simulink model "UAV_sync_unknown_sim"  (R2018b)
settings: Solver=ode23tb  StartTime=0.0  StopTime=35  RelTol=1e-3
values from neighbouring files (symbols this model uses):
  Bm = [zeros(6,6); eye(6)]    [UAV_sync_unknown.m]    (also in UAV_sync_unknown_gap.m)
  C_rho = 1.225    [SC42120_UAV_Preconditions.m]
  D0 = [M0 0 0 0 0 0 ... (first row only)    [SC42120_UAV_Preconditions.m]
  Derivative_gain_phi = 50    [SC42120_UAV_Preconditions.m]
  Derivative_gain_psi = 50    [SC42120_UAV_Preconditions.m]
  Derivative_gain_theta = 50    [SC42120_UAV_Preconditions.m]
  Derivative_gain_x = 50    [SC42120_UAV_Preconditions.m]
  Derivative_gain_y = 50    [SC42120_UAV_Preconditions.m]
  Derivative_gain_z = 50    [SC42120_UAV_Preconditions.m]
  G = 9.80665    [SC42120_UAV_Preconditions.m]
  g0 = [0;0;-M0*G;0;0;0]    [SC42120_UAV_Preconditions.m]
  I0 = [0.02 0 -0.01 ... (first row only)    [SC42120_UAV_Preconditions.m]
  InitWind = [0;0;0]    [SC42120_UAV_Preconditions.m]
  Kp = diag(P)    [SC42120_UAV_Preconditions.m]
  Kv = diag(V)    [SC42120_UAV_Preconditions.m]
  M0 = 10    [SC42120_UAV_Preconditions.m]
  M1 = 20    [UAV_sync_known.m]    (also in UAV_sync_unknown.m; UAV_sync_unknown_gap.m)
  M2 = 30    [UAV_sync_known.m]    (also in UAV_sync_unknown.m; UAV_sync_unknown_gap.m)
  M3 = 40    [UAV_sync_known.m]    (also in UAV_sync_unknown.m; UAV_sync_unknown_gap.m)
  M4 = 50    [UAV_sync_known.m]    (also in UAV_sync_unknown.m; UAV_sync_unknown_gap.m)
  P = [Proportional_x Proportional_y Proportional_z Proportional_phi Proportional_theta Proportional_psi]    [SC42120_UAV_Preconditions.m]    (also in UAV_sync_unknown.m = lyap(Am',Q); UAV_sync_unknown_gap.m = lyap(Am',Q); drawDATCOMaircraft.m = temparray)
  Proportional_phi = 50    [SC42120_UAV_Preconditions.m]
  Proportional_psi = 50    [SC42120_UAV_Preconditions.m]
  Proportional_theta = 50    [SC42120_UAV_Preconditions.m]
  Proportional_x = 50    [SC42120_UAV_Preconditions.m]
  Proportional_y = 50    [SC42120_UAV_Preconditions.m]
  Proportional_z = 50    [SC42120_UAV_Preconditions.m]
undefined symbols (not defined in the file or in its folder): Aero, APlane, Bxl, C, Ctr, deg, DiscIntNeverNeededParam, F, Guid, Init, Light, MIL, Path, rad, s, Trim, Utility
libraries: aerolibconvert2 x37, sharedutil x18, simulink x15, dspsigops x7, shared6dof x6, aerolibasang x4, simulink_extras x3, aerolibadyn x1, aerolibtransform2 x1, aerolibwind2 x1
(part 3 of 7)

== system UAV_sync_unknown_sim/Node 0/VF Approach/AUTOPILOT/Navigation Controller ==
  note: Activate bias only if you have troubles with undesired settling orbits.
  ReferenceCourse : Inport  Unit=deg
  DerCond : Inport  Port=2
  Angle Conversion : aerolibconvert2/Angle Conversion  IU=rad  OU=deg
  Bias : Bias  Bias=360
  Bus Selector : BusSelector  OutputSignals=Course
  Constant : Constant  Value=45
  Discrete PID Controller : simulink/Continuous/PID Controller  Controller=PD  Form=Parallel  TimeDomain=Discrete-time  SampleTime=Ctr.TS  IntegratorMethod=Forward Euler  FilterMethod=Forward Euler  ControllerParametersSource=internal  P=Ctr.Hdg2Roll.NAV_ROLL_P  I=0.01  D=Ctr.Hdg2Roll.NAV_ROLL_D  UseFilter=on  N=2*pi*20  TunerSelectOption=Transfer Function Based (PID Tuner App)  InitialConditionSource=internal  InitialConditionForIntegrator=0  InitialConditionForFilter=0  DifferentiatorICPrevScaledInput=0  ExternalReset=none  TrackingMode=off  Kt=1  LimitOutput=on  UpperSaturationLimit=45  LowerSaturationLimit=-45  LinearizeAsGain=off  AntiWindupMode=clamping  Kb=1  POutMin=[]  POutMax=[]  IOutMin=[]  IOutMax=[]  DOutMin=[]  DOutMax=[]  NOutMin=[]  NOutMax=[]  SumOutMin=[]  SumOutMax=[]  SaturationOutMin=[]  SaturationOutMax=[]  PParamMin=[]  PParamMax=[]  IParamMin=[]  IParamMax=[]  DParamMin=[]  DParamMax=[]  NParamMin=[]  NParamMax=[]  KbParamMin=[]  KbParamMax=[]  KtParamMin=[]  KtParamMax=[]  KbOutMin=[]  KbOutMax=[]  KtOutMin=[]  KtOutMax=[]  IntegratorOutMin=[]  IntegratorOutMax=[]  FilterOutMin=[]  FilterOutMax=[]  SumI1OutMin=[]  SumI1OutMax=[]  SumI2OutMin=[]  SumI2OutMax=[]  SumI3OutMin=[]  SumI3OutMax=[]  SumI4OutMin=[]  SumI4OutMax=[]  SumDOutMin=[]  SumDOutMax=[]  DifferentiatorOutMin=[]  DifferentiatorOutMax=[]  FilterDiffOutCoefMin=[]  FilterDiffOutCoefMax=[]  ReciprocalOutMin=[]  ReciprocalOutMax=[]  SumDenOutMin=[]  SumDenOutMax=[]  SumNumOutMin=[]  SumNumOutMax=[]  DivideOutMin=[]  DivideOutMax=[]  IntegratorContinuousStateAttributes=''  IntegratorStateMustResolveToSignalObject=off  IntegratorRTWStateStorageClass=Auto  FilterContinuousStateAttributes=''  FilterStateMustResolveToSignalObject=off  FilterRTWStateStorageClass=Auto  ParallelPVariant=InternalParameters  IdealPVariant=Disabled  IVariant=Disabled  DVariant=InternalParameters  IntegratorVariant=Disabled  SatVariant=Enabled  AWVariant=Disabled  PCopyVariant=Disabled  TRVariant=Disabled  FdbkBlocksVariant=Forward  IdealPFdbkVariant=Disabled  SatFdbkVariant=Disabled  DerivativeFilterVariant=ForwardEulerFilter  NVariant=InternalParameters  NCopyVariant=Disabled  FilterICVariant=InternalICsFilter  IntegratorICVariant=Disabled  ExternalResetVariant=Disabled  TRSumVariant=Passthrough  SumFdbkVariant=Disabled  SumVariant=Sum_PD
  Manual Switch : ManualSwitch  CurrentSetting=0
  Manual Switch1 : ManualSwitch
  PID : Subsystem  Commented=on
  Scope : Scope
  Scope1 : Scope
  Scope2 : Scope  NumInputPorts=2
  Step : Step  Time=10  After=90  SampleTime=0
  Sum : Sum  Inputs=|+-
  Unwrap : Subsystem
  Unwrap1 : dspsigops/Unwrap  tol=pi  InputProcessing=Columns as channels (frame based)  running=off
  Zero-Order Hold : ZeroOrderHold  SampleTime=1/400
  BankAngle : Outport  Unit=deg
  wires:
  Bus Selector/1 -> Unwrap1/1  "<Course>"
  Discrete PID Controller/1 -> Manual Switch1/1, Scope/1
  DerCond/1 -> Bus Selector/1
  Unwrap1/1 -> Angle Conversion/1  "chi_measured"
  Sum/1 -> Scope1/1, Discrete PID Controller/1
  Angle Conversion/1 -> Sum/2, Scope2/2
  ReferenceCourse/1 -> Manual Switch/2
  Unwrap/1(Out) -> Scope2/1, Sum/1
  Manual Switch/1 -> Bias/1
  Step/1 -> Zero-Order Hold/1
  Zero-Order Hold/1 -> Manual Switch/1
  Manual Switch1/1 -> BankAngle/1
  Constant/1 -> Manual Switch1/2
  Bias/1 -> Unwrap/1(In)

== system UAV_sync_unknown_sim/Node 0/VF Approach/AUTOPILOT/Total Energy Control System ==
  note: TECS (Total Energy Control System)
      |
      | It is meant to solve the cross-coupling between height and airspeed control. This is a simplified version of the TECS (see thesis for details). This implementation has the same theoretical behaviour of ArduPilot, but without a direct correspondence with its parameters.
  PlantData : Inport
  Target_Height : Inport  Port=2
  Target_Airspeed : Inport  Port=3
  Bus Selector1 : BusSelector  OutputSignals=xyh
  Discrete PID Controller 1 : simulink/Continuous/PID Controller  Controller=PID  Form=Parallel  TimeDomain=Discrete-time  SampleTime=Ctr.TS  IntegratorMethod=Forward Euler  FilterMethod=Forward Euler  ControllerParametersSource=internal  P=1.73635676332661  I=0.34363794334664  D=0.534286386520939  UseFilter=on  N=1.11842208231346  TunerSelectOption=Transfer Function Based (PID Tuner App)  InitialConditionSource=internal  InitialConditionForIntegrator=0  InitialConditionForFilter=0  DifferentiatorICPrevScaledInput=0  ExternalReset=none  TrackingMode=off  Kt=1  LimitOutput=on  UpperSaturationLimit=100  LowerSaturationLimit=0  LinearizeAsGain=off  AntiWindupMode=clamping  Kb=1  POutMin=[]  POutMax=[]  IOutMin=[]  IOutMax=[]  DOutMin=[]  DOutMax=[]  NOutMin=[]  NOutMax=[]  SumOutMin=[]  SumOutMax=[]  SaturationOutMin=[]  SaturationOutMax=[]  PParamMin=[]  PParamMax=[]  IParamMin=[]  IParamMax=[]  DParamMin=[]  DParamMax=[]  NParamMin=[]  NParamMax=[]  KbParamMin=[]  KbParamMax=[]  KtParamMin=[]  KtParamMax=[]  KbOutMin=[]  KbOutMax=[]  KtOutMin=[]  KtOutMax=[]  IntegratorOutMin=[]  IntegratorOutMax=[]  FilterOutMin=[]  FilterOutMax=[]  SumI1OutMin=[]  SumI1OutMax=[]  SumI2OutMin=[]  SumI2OutMax=[]  SumI3OutMin=[]  SumI3OutMax=[]  SumI4OutMin=[]  SumI4OutMax=[]  SumDOutMin=[]  SumDOutMax=[]  DifferentiatorOutMin=[]  DifferentiatorOutMax=[]  FilterDiffOutCoefMin=[]  FilterDiffOutCoefMax=[]  ReciprocalOutMin=[]  ReciprocalOutMax=[]  SumDenOutMin=[]  SumDenOutMax=[]  SumNumOutMin=[]  SumNumOutMax=[]  DivideOutMin=[]  DivideOutMax=[]  IntegratorContinuousStateAttributes=''  IntegratorStateMustResolveToSignalObject=off  IntegratorRTWStateStorageClass=Auto  FilterContinuousStateAttributes=''  FilterStateMustResolveToSignalObject=off  FilterRTWStateStorageClass=Auto  ParallelPVariant=InternalParameters  IdealPVariant=Disabled  IVariant=InternalParameters  DVariant=InternalParameters  IntegratorVariant=Discrete  SatVariant=Enabled  AWVariant=DiscClampingParallel  PCopyVariant=Disabled  TRVariant=Disabled  FdbkBlocksVariant=Forward  IdealPFdbkVariant=Disabled  SatFdbkVariant=Disabled  DerivativeFilterVariant=ForwardEulerFilter  NVariant=InternalParameters  NCopyVariant=Disabled  FilterICVariant=InternalICsFilter  IntegratorICVariant=InternalICs  ExternalResetVariant=Disabled  TRSumVariant=Passthrough  SumFdbkVariant=Disabled  SumVariant=Sum_PID
  Discrete PID Controller 2 : simulink/Continuous/PID Controller  Controller=PID  Form=Parallel  TimeDomain=Discrete-time  SampleTime=Ctr.TS  IntegratorMethod=Forward Euler  FilterMethod=Forward Euler  ControllerParametersSource=internal  P=0.0957032759552278  I=0.0036993820124705  D=0.00128202697815644  UseFilter=on  N=46.36307138661  TunerSelectOption=Transfer Function Based (PID Tuner App)  InitialConditionSource=internal  InitialConditionForIntegrator=0  InitialConditionForFilter=0  DifferentiatorICPrevScaledInput=0  ExternalReset=none  TrackingMode=off  Kt=1  LimitOutput=on  UpperSaturationLimit=30  LowerSaturationLimit=-30  LinearizeAsGain=off  AntiWindupMode=clamping  Kb=1  POutMin=[]  POutMax=[]  IOutMin=[]  IOutMax=[]  DOutMin=[]  DOutMax=[]  NOutMin=[]  NOutMax=[]  SumOutMin=[]  SumOutMax=[]  SaturationOutMin=[]  SaturationOutMax=[]  PParamMin=[]  PParamMax=[]  IParamMin=[]  IParamMax=[]  DParamMin=[]  DParamMax=[]  NParamMin=[]  NParamMax=[]  KbParamMin=[]  KbParamMax=[]  KtParamMin=[]  KtParamMax=[]  KbOutMin=[]  KbOutMax=[]  KtOutMin=[]  KtOutMax=[]  IntegratorOutMin=[]  IntegratorOutMax=[]  FilterOutMin=[]  FilterOutMax=[]  SumI1OutMin=[]  SumI1OutMax=[]  SumI2OutMin=[]  SumI2OutMax=[]  SumI3OutMin=[]  SumI3OutMax=[]  SumI4OutMin=[]  SumI4OutMax=[]  SumDOutMin=[]  SumDOutMax=[]  DifferentiatorOutMin=[]  DifferentiatorOutMax=[]  FilterDiffOutCoefMin=[]  FilterDiffOutCoefMax=[]  ReciprocalOutMin=[]  ReciprocalOutMax=[]  SumDenOutMin=[]  SumDenOutMax=[]  SumNumOutMin=[]  SumNumOutMax=[]  DivideOutMin=[]  DivideOutMax=[]  IntegratorContinuousStateAttributes=''  IntegratorStateMustResolveToSignalObject=off  IntegratorRTWStateStorageClass=Auto  FilterContinuousStateAttributes=''  FilterStateMustResolveToSignalObject=off  FilterRTWStateStorageClass=Auto  ParallelPVariant=InternalParameters  IdealPVariant=Disabled  IVariant=InternalParameters  DVariant=InternalParameters  IntegratorVariant=Discrete  SatVariant=Enabled  AWVariant=DiscClampingParallel  PCopyVariant=Disabled  TRVariant=Disabled  FdbkBlocksVariant=Forward  IdealPFdbkVariant=Disabled  SatFdbkVariant=Disabled  DerivativeFilterVariant=ForwardEulerFilter  NVariant=InternalParameters  NCopyVariant=Disabled  FilterICVariant=InternalICsFilter  IntegratorICVariant=InternalICs  ExternalResetVariant=Disabled  TRSumVariant=Passthrough  SumFdbkVariant=Disabled  SumVariant=Sum_PID
  Fcn2 : Fcn  Expr=0.5 * u(1)^2
  Fcn4 : Fcn  Expr=0.5 * u(1)^2
  Gain1 : Gain  Gain=C.g
  Gain3 : Gain  Gain=C.g
  Selector1 : Selector  InputPortWidth=3  IndexOptions=Index vector (dialog)  Indices=3  OutputSizes=1
  Sum : Sum  Inputs=|++
  Sum11 : Sum  Inputs=+-
  Sum12 : Sum  Inputs=+-
  Sum13 : Sum  Inputs=|-+
  Sum8 : Sum  Inputs=|++
  Sum9 : Sum  Inputs=|-+
  ThrottleDem : Outport
  PitchDem : Outport  Port=2
  wires:
  Discrete PID Controller 2/1 -> PitchDem/1  "pitch"
  Discrete PID Controller 1/1 -> ThrottleDem/1  "throttle"
  [Va] -> Fcn2/1
  Fcn2/1 -> Sum/2, Sum11/2  "SKE"
  PlantData/1 -> Bus Selector1/1
  Bus Selector1/1 -> Selector1/1  "<xyh>"
  Selector1/1 -> Gain1/1
  Gain1/1 -> Sum/1, Sum11/1  "SPE"
  Target_Height/1 -> Gain3/1
  Gain3/1 -> Sum12/1, Sum8/1  "SPE_c"
  Target_Airspeed/1 -> Fcn4/1
  Fcn4/1 -> Sum12/2, Sum8/2  "SKE_c"
  Sum/1 -> Sum9/1  "Specific total energy"
  Sum8/1 -> Sum9/2  "Demanded specific total energy"
  Sum9/1 -> Discrete PID Controller 1/1  "STE err"
  Sum11/1 -> Sum13/1  "Specific energy balance"
  Sum12/1 -> Sum13/2  "Demanded specific energy balance"
  Sum13/1 -> Discrete PID Controller 2/1  "SBE err"

== system UAV_sync_unknown_sim/Node 0/VF Approach/BIXLER DYNAMICS/Actuator Dynamics ==
  In : Inport
  +-15 : Saturate  UpperLimit=15  LowerLimit=-15
  +-25 : Saturate  UpperLimit=25  LowerLimit=-25
  +-30 : Saturate  UpperLimit=30  LowerLimit=-30
  Bus Creator1 : BusCreator  Inputs='delta_ail','delta_elev','delta_rudd'
  Bus Selector : BusSelector  OutputSignals=ailerons,elevator,rudder
  Scope : Scope  NumInputPorts=2
  Transfer Fcn : TransferFcn  Numerator=[45]  Denominator=[1 45]
  Transfer Fcn1 : TransferFcn  Numerator=[45]  Denominator=[1 45]
  Transfer Fcn2 : TransferFcn  Numerator=[45]  Denominator=[1 45]
  Out : Outport  Unit=deg
  wires:
  +-30/1 -> Bus Creator1/1  "delta_ail"
  Bus Creator1/1 -> Out/1  "ControlActions"
  +-25/1 -> Bus Creator1/3  "delta_rudd"
  +-15/1 -> Bus Creator1/2  "delta_elev"
  Bus Selector/2 -> Transfer Fcn1/1  "<elevator>"
  Bus Selector/1 -> Scope/1, Transfer Fcn/1  "<ailerons>"
  Bus Selector/3 -> Transfer Fcn2/1  "<rudder>"
  In/1 -> Bus Selector/1
  Transfer Fcn/1 -> Scope/2, +-30/1
  Transfer Fcn1/1 -> +-15/1
  Transfer Fcn2/1 -> +-25/1

== system UAV_sync_unknown_sim/Node 0/VF Approach/BIXLER DYNAMICS/Derived Conditions ==
  note: WAE = Wind Angle Error
  EnvData : Inport
  PlantData : Inport  Port=2
  Angle Conversion : aerolibconvert2/Angle Conversion  IU=rad  OU=deg
  Bus Selector : BusSelector  OutputSignals=Wind total (body)
  Bus Selector1 : BusSelector  OutputSignals=Velocity (body),Velocity (inertial)
  Bus Selector2 : BusSelector  OutputSignals=Euler angles (rad)
  Constant : Constant  Value=C.rho
  Dynamic Pressure : aerolibasang/Dynamic Pressure
  "Incidence, Sideslip, & Airspeed" : aerolibasang/Incidence, Sideslip, & Airspeed
      settings: SourceProductName=Aerospace Blockset
  Scope : Scope
  Selector : Selector  InputPortWidth=3  IndexOptions=Index vector (dialog)  Indices=3  OutputSizes=1
  Selector1 : Selector  InputPortWidth=3  IndexOptions=Index vector (dialog)  Indices=2  OutputSizes=1
  Selector3 : Selector  InputPortWidth=3  IndexOptions=Index vector (dialog)  Indices=1  OutputSizes=1
  Sum2 : Sum  Inputs=|-+
  Sum4 : Sum  Inputs=+-|
  Sum5 : Sum  Inputs=+-|
  Trigonometric Function1 : Trigonometry  Operator=atan2
  qbar : Outport  Unit=kg/m/s^2
  alpha : Outport  Port=2  Unit=rad
  beta : Outport  Port=3  Unit=rad
  Va : Outport  Port=4  Unit=m/s
  CourseAngle : Outport  Port=5  Unit=rad
  CrabAngle : Outport  Port=6  Unit=rad
  WAE : Outport  Port=7  Unit=rad
  wires:
  Dynamic Pressure/1 -> qbar/1
  Bus Selector1/1 -> Sum2/2, Dynamic Pressure/1  "<Velocity (body)>"
  "Incidence, Sideslip, & Airspeed"/2 -> [beta], beta/1
  "Incidence, Sideslip, & Airspeed"/3 -> Va/1
  Bus Selector/1 -> Sum2/1  "<Wind total (body)>"
  EnvData/1 -> Bus Selector/1
  Constant/1 -> Dynamic Pressure/2
  Sum2/1 -> "Incidence, Sideslip, & Airspeed"/1  "V_a_vector"
  "Incidence, Sideslip, & Airspeed"/1 -> alpha/1
  PlantData/1 -> Bus Selector2/1, Bus Selector1/1
  Bus Selector2/1 -> Selector/1  "<Euler angles (rad)>"
  Selector/1 -> Sum4/2  "psi"
  Selector1/1 -> Trigonometric Function1/1  "V_gy"
  Bus Selector1/2 -> Selector3/1, Selector1/1  "<Velocity (inertial)>"
  Sum4/1 -> Sum5/1, CrabAngle/1
  Sum5/1 -> WAE/1
  [beta] -> Sum5/2
  Selector3/1 -> Trigonometric Function1/2  "V_gx"
  Trigonometric Function1/1 -> Sum4/1, CourseAngle/1, Angle Conversion/1
  Angle Conversion/1 -> Scope/1

== system UAV_sync_unknown_sim/Node 0/VF Approach/BIXLER DYNAMICS/RUBBISH BIN ==
  Angle Conversion1 : aerolibconvert2/Angle Conversion  Commented=on  IU=deg  OU=rad
  Clock : Clock  Commented=on
  Constant1 : Constant  Commented=on  Value=0
  From1 : From  Commented=on  GotoTag=throttle
  From2 : From  Commented=on  GotoTag=Target_Height  TagVisibility=global
  From3 : From  Commented=on  GotoTag=Target_Airspeed  TagVisibility=global
  From7 : From  Commented=on  GotoTag=throttle
  From9 : From  Commented=on  GotoTag=PlantData
  Orbit : Subsystem  Commented=on
  Reference Signals : Subsystem  Commented=on
  Reference Signals1 : Subsystem  Commented=on
  Straight Line : Subsystem  Commented=on
  Switch : Switch  Commented=on  Criteria=u2 > Threshold  Threshold=50
  TECS : Subsystem  Commented=on
  Vector Field : MATLAB Function  Commented=on  TreatAsAtomicUnit=on
  wires:
  From7/1 -> Reference Signals/1(Throttle)
  Clock/1 -> Switch/2
  Constant1/1 -> Angle Conversion1/1
  Angle Conversion1/1 -> Switch/3
  Vector Field/1(y) -> Switch/1
  From1/1 -> Reference Signals1/1(Throttle)
  From2/1 -> TECS/3(HeightDemand)
  From3/1 -> TECS/2(TAS_dem)
  From9/1 -> TECS/1(PlantData)

== system UAV_sync_unknown_sim/Node 0/VF Approach/BIXLER DYNAMICS/Sampling ==
  Cont. : Inport
  Bus Creator : BusCreator  Inputs=3
  Zero-Order Hold : ZeroOrderHold  SampleTime=1/400
  Zero-Order Hold1 : ZeroOrderHold  SampleTime=1/10
  Cont.+Disc. : Outport
  wires:
  Cont./1 -> Zero-Order Hold1/1, Zero-Order Hold/1, Bus Creator/3  "PlantData"
  Bus Creator/1 -> Cont.+Disc./1
  Zero-Order Hold1/1 -> Bus Creator/2  "PlantData @10Hz"
  Zero-Order Hold/1 -> Bus Creator/1  "PlantData @400Hz"

== system UAV_sync_unknown_sim/Node 0/VF Approach/BIXLER DYNAMICS/Sampling  ==
  Cont. : Inport
  Bus Creator : BusCreator  Inputs=3
  Zero-Order Hold : ZeroOrderHold  SampleTime=1/400
  Zero-Order Hold1 : ZeroOrderHold  SampleTime=1/10
  Cont.+Disc. : Outport
  wires:
  Zero-Order Hold/1 -> Bus Creator/1  "DerCond @400Hz"
  Zero-Order Hold1/1 -> Bus Creator/2  "DerCond @10Hz"
  Bus Creator/1 -> Cont.+Disc./1
  Cont./1 -> Bus Creator/3, Zero-Order Hold/1, Zero-Order Hold1/1  "DerCond"

== system UAV_sync_unknown_sim/Node 0/VF Approach/BIXLER DYNAMICS/Throttle Dynamics ==
  In : Inport  Unit=%
  0-100 : Saturate  UpperLimit=100  LowerLimit=0
  Transfer Fcn2 : TransferFcn  Numerator=[45]  Denominator=[1 45]
  Out : Outport  Unit=%
  wires:
  In/1 -> Transfer Fcn2/1
  0-100/1 -> Out/1
  Transfer Fcn2/1 -> 0-100/1

== system UAV_sync_unknown_sim/Node 0/VF Approach/BIXLER DYNAMICS/Vehicle Airframe ==
  Throttle_cmd : Inport  Unit=%
  ControlActions : Inport  Port=2
  DerCond : Inport  Port=3
  6DOF (Euler Angles) : shared6dof/6DOF (Euler Angles)  units=Metric (MKS)  mtype=Fixed  rep=Euler Angles  xme_0=Init.xyz  Vm_0=Init.uvw  eul_0=deg2rad(Init.attitude)  pm_0=deg2rad(Init.pqr)  mass_0=Bxl.mass  mass_e=0.5  mass_f=2.0  inertia=Bxl.J  inertia_e=eye(3)  inertia_f=2*eye(3)  k_quat=1.0  vre_flag=on  abi_flag=off  aMode=aMode  xme_statename=''  Vm_statename=''  eul_statename=''  quat_statename=''  pm_statename=''  mass_statename=''
      settings: SourceProductBaseCode=AE
  Aerodynamics : Subsystem
  Bus Creator : BusCreator  Inputs=Velocity (inertial),Position (inertial),xyh,Euler angles (rad),ome_e,Angular rates (body) (rad/s),From inertial to body matrix,Velocity (body),Angular accelerations (body/body),Accelerations (body/body),xyh_body
  "DerCond " : InportShadow  Port=3
  Gain : Gain  Gain=[1 1 -1]
  Gravity Force : Subsystem
  Product : Product  Multiplication=Matrix(*)
  Propulsion : Subsystem
  Sum : Sum
  Sum1 : Sum  Inputs=+++|
  to Omega_e : Subsystem
  PlantData : Outport
  wires:
  [DCM] -> Product/1, Bus Creator/7  "From inertial to body matrix"
  [euler] -> Bus Creator/4, to Omega_e/1(euler)  "Euler angles (rad)"
  [Vb] -> Bus Creator/8  "Velocity (body)"
  [PlantData] -> Aerodynamics/1(PlantData)
  [Ve] -> Bus Creator/1  "Velocity (inertial)"
  [Xe] -> Gain/1, Bus Creator/2  "Position (inertial)"
  [A_b] -> Bus Creator/10  "Accelerations (body/body)"
  ControlActions/1 -> Aerodynamics/3(Control)
  Sum1/1 -> 6DOF (Euler Angles)/1
  Bus Creator/1 -> PlantData/1, [PlantData]
  Sum/1 -> 6DOF (Euler Angles)/2
  [PlantData] -> Gravity Force/1(PlantData)
  Gravity Force/1(Fg) -> Sum1/1
  Throttle_cmd/1 -> Propulsion/1(Throttle)
  Propulsion/2(M) -> Sum/1
  Propulsion/1(F) -> Sum1/2
  "DerCond "/1 -> Aerodynamics/2(DerCond)
  Aerodynamics/1(AeroForces) -> Sum1/3
  Aerodynamics/2(AeroMoments) -> Sum/2
  [ome_d_b] -> Bus Creator/9  "Angular accelerations (body/body)"
  [ome_b] -> Bus Creator/6, to Omega_e/2(ome_b)  "Angular rates (body) (rad/s)"
  Gain/1 -> Product/2, Bus Creator/3  "xyh"
  to Omega_e/1(ome_e) -> Bus Creator/5  "ome_e"
  6DOF (Euler Angles)/1 -> [Ve]
  6DOF (Euler Angles)/2 -> [Xe]
  6DOF (Euler Angles)/3 -> [euler]
  6DOF (Euler Angles)/4 -> [DCM]
  6DOF (Euler Angles)/5 -> [Vb]
  6DOF (Euler Angles)/6 -> [ome_b]
  6DOF (Euler Angles)/7 -> [ome_d_b]
  6DOF (Euler Angles)/8 -> [A_b]
  DerCond/1 -> Propulsion/2(DerCond)
  Product/1 -> Bus Creator/11  "xyh_body"

== system UAV_sync_unknown_sim/Node 0/VF Approach/ENVIRONMENT/Slowly time varying wind gen. ==
  Constant : Constant  Value=0
  Fcn : Fcn  Expr=u(1)*cos(u(2))
  Fcn1 : Fcn  Expr=u(1)*sin(u(2))
  Mux : Mux  Inputs=2
  Mux1 : Mux  Inputs=3
  Sine Wave : Sin  Amplitude=3  Frequency=0.01  SampleTime=0
  Sine Wave1 : Sin  Amplitude=pi  Frequency=0.01  SampleTime=0
  Out1 : Outport
  wires:
  Fcn/1 -> Mux1/1
  Mux1/1 -> Out1/1
  Constant/1 -> Mux1/3
  Sine Wave1/1 -> Mux/2
  Sine Wave/1 -> Mux/1
  Fcn1/1 -> Mux1/2
  Mux/1 -> Fcn1/1, Fcn/1

== system UAV_sync_unknown_sim/Node 0/VF Approach/MANUAL INPUTS/Trim conditions ==
  note: Trim condition on/off. (default: off)
      |
      | Reminder:
      | if on, Manual Control switches must be up.
  throttle : Inport
  ail : Inport  Port=2
  elev : Inport  Port=3
  rudd : Inport  Port=4
  Manual Switch{,1..3} (4 alike) : ManualSwitch  CurrentSetting=0
  Manual_cmd1 : Constant  Value=Trim.throttle
  Manual_cmd2 : Constant  Value=Trim.ail
  Manual_cmd3 : Constant  Value=Trim.elev
  Manual_cmd7 : Constant  Value=Trim.rudd
  throttout : Outport  Unit=%
  ailout : Outport  Port=2  Unit=deg
  elevout : Outport  Port=3  Unit=deg
  ruddout : Outport  Port=4  Unit=deg
  wires:
  throttle/1 -> Manual Switch/2
  Manual_cmd1/1 -> Manual Switch/1
  Manual_cmd2/1 -> Manual Switch1/1
  Manual_cmd3/1 -> Manual Switch2/1
  Manual_cmd7/1 -> Manual Switch3/1
  ail/1 -> Manual Switch1/2
  rudd/1 -> Manual Switch3/2
  Manual Switch/1 -> throttout/1
  Manual Switch1/1 -> ailout/1
  Manual Switch2/1 -> elevout/1
  Manual Switch3/1 -> ruddout/1
  elev/1 -> Manual Switch2/2

== system UAV_sync_unknown_sim/Node 0/VF Approach/PATH FOLLOWING/Extract Vg ==
  PlantData : Inport
  EnvData : Inport  Port=2
  10Hz : ZeroOrderHold  Commented=through  SampleTime=1/10
  "10Hz " : ZeroOrderHold  SampleTime=1/10
  Bus Selector1 : BusSelector  OutputSignals=Velocity (body)
  Bus Selector4 : BusSelector  OutputSignals=Wind velocity (dyn) (body)
  Dot Product1 : DotProduct  InputSameDT=on  OutDataTypeStr=Inherit: Inherit via internal rule
  Selector : Selector  InputPortWidth=3  IndexOptions=Index vector (dialog)  Indices=[1 2]  OutputSizes=1
  Sqrt1 : Sqrt  SaturateOnIntegerOverflow=on
  Sum2 : Sum  Inputs=|+-
  Vg : Outport
  wires:
  PlantData/1 -> Bus Selector1/1
  EnvData/1 -> 10Hz/1
  Bus Selector1/1 -> Sum2/1  "<Velocity (body)>"
  Bus Selector4/1 -> Sum2/2  "<Wind velocity (dyn) (body)>"
  Sum2/1 -> Selector/1  "Vg"
  Selector/1 -> Dot Product1/2, Dot Product1/1  "Vg_xy"
  Dot Product1/1 -> Sqrt1/1
  Sqrt1/1 -> "10Hz "/1
  "10Hz "/1 -> Vg/1
  10Hz/1 -> Bus Selector4/1

== system UAV_sync_unknown_sim/Node 0/VF Approach/PATH FOLLOWING/Extract Vg_prime ==
  PlantData : Inport
  Bus Selector6 : BusSelector  OutputSignals=Velocity (body)
  Dot Product : DotProduct  InputSameDT=on  OutDataTypeStr=Inherit: Inherit via internal rule
  Selector : Selector  InputPortWidth=3  IndexOptions=Index vector (dialog)  Indices=[1 2]  OutputSizes=1
  Sqrt : Sqrt  SaturateOnIntegerOverflow=on
  Zero-Order Hold : ZeroOrderHold  SampleTime=1/10
  Vg' : Outport
  wires:
  Sqrt/1 -> Zero-Order Hold/1  "Vg'"
  PlantData/1 -> Bus Selector6/1
  Bus Selector6/1 -> Selector/1  "<Velocity (body)>"
  Dot Product/1 -> Sqrt/1
  Selector/1 -> Dot Product/2, Dot Product/1
  Zero-Order Hold/1 -> Vg'/1

== system UAV_sync_unknown_sim/Node 0/VF Approach/PATH FOLLOWING/Orbit Path Following (Enabled Subsystem) ==
  note: Out
  note: 3. Controller
  note: 2. Desired Course (chi_d)
  note: 1. Gamma computation
  note: Vg' estimator
  PlantData : Inport
  DerCond : Inport  Port=2
  GuidData : Inport  Port=3
  Vg : Inport  Port=4
  Vg_prime : Inport  Port=5
  Enable : EnablePort  StatesWhenEnabling=reset  PropagateVarSize=During execution
  10 Hz : ZeroOrderHold  SampleTime=1/10
  "10 Hz " : ZeroOrderHold  SampleTime=1/10
  Bus Selector1 : BusSelector  OutputSignals=Position (inertial)
  Bus Selector5 : BusSelector  OutputSignals=Course
  Bus Selector7 : BusSelector  OutputSignals=Orbit_C,Orbit_R,Orbit_j
  Chi_d : Subsystem
  Compute gamma and distance to center : Subsystem
  "DerCond " : InportShadow  Port=2
  Goto Tag Visibility 1 : GotoTagVisibility  GotoTag=j
  Goto Tag Visibility 2 : GotoTagVisibility  GotoTag=R
  Goto Tag Visibility 3 : GotoTagVisibility  GotoTag=C
  Goto Tag Visibility 4 : GotoTagVisibility  GotoTag=Vg_prime
  Loiter Controller : Subsystem
  Selector1 : Selector  InputPortWidth=3  IndexOptions=Index vector (dialog)  Indices=[1 2]  OutputSizes=1
  Unwrap : dspsigops/Unwrap  tol=pi  running=off
  Vg Estimator : Subsystem
  Vg. : InportShadow  Port=4
  chi_c_O : Outport
  Vg_hat_O : Outport  Port=2
  chi_d_O : Outport  Port=3
  d_tilde : Outport  Port=4
  tag scope: C=scoped, R=scoped, Vg_prime=scoped, j=scoped
  wires:
  Compute gamma and distance to center/1(gamma) -> [gamma]
  [Vg_hat] -> Vg_hat_O/1  "Vg_hat"
  [chi_d] -> chi_d_O/1  "chi_d_O"
  [chi_c] -> chi_c_O/1  "chi_c_O"
  Bus Selector1/1 -> Selector1/1  "<Position (inertial)>"
  Selector1/1 -> 10 Hz/1
  Compute gamma and distance to center/2(d) -> [d]
  [xy] -> Compute gamma and distance to center/1(xy)
  [gamma] -> Chi_d/1(gamma)
  [j] -> Chi_d/2(j)
  [d] -> Chi_d/3(d)
  [R] -> Chi_d/4(r)
  Chi_d/1(chi_d) -> [chi_d]
  Chi_d/2(d_tilde) -> [d_tilde]
  [chi_meas] -> Vg Estimator/1(chi)
  [d] -> Vg Estimator/2(d)
  [gamma] -> Vg Estimator/3(gamma)
  [chi_d] -> Vg Estimator/4(chi_d)
  Vg Estimator/1(Vg_hat) -> [Vg_hat]
  [chi_meas] -> Loiter Controller/1(chi)
  [chi_d] -> Loiter Controller/2(chi_d)
  [d] -> Loiter Controller/3(d)
  [Vg_hat] -> Loiter Controller/4(Vg_hat)
  [gamma] -> Loiter Controller/5(gamma)
  Loiter Controller/1(chi_c) -> [chi_c]
  DerCond/1 -> Bus Selector5/1
  "10 Hz "/1 -> Unwrap/1
  Unwrap/1 -> [chi_meas]
  [C] -> Compute gamma and distance to center/2(OrbitCenter)
  PlantData/1 -> Bus Selector1/1
  Bus Selector5/1 -> "10 Hz "/1  "<Course>"
  Vg./1 -> Loiter Controller/6(Vg)
  Vg/1 -> Vg Estimator/5(vg)
  GuidData/1 -> Bus Selector7/1
  Bus Selector7/3 -> [j]  "<Orbit_j>"
  Bus Selector7/2 -> [R]  "<Orbit_R>"
  Bus Selector7/1 -> [C]  "<Orbit_C>"
  [d_tilde] -> d_tilde/1  "d_tilde"
  Vg_prime/1 -> [Vg_prime]
  "DerCond "/1 -> Vg Estimator/6(DerCond)
  10 Hz/1 -> [xy]
  [chi_meas] -> Compute gamma and distance to center/3(chi)

== system UAV_sync_unknown_sim/Node 0/VF Approach/PATH FOLLOWING/Straight-line Path Following (Enabled Subsystem) ==
  note: Out
  note: 3. Controller
  note: Vg' estimator
  note: 2. Desired Course (chi_d as function of e_y)
  note: 1. Crosstrack error computation
  PlantData : Inport
  DerCond : Inport  Port=2
  GuidData : Inport  Port=3
  Vg : Inport  Port=4
  Vg_prime : Inport  Port=5
  Enable : EnablePort  StatesWhenEnabling=reset  PropagateVarSize=During execution
  10 Hz : ZeroOrderHold  SampleTime=1/10
  "10 Hz " : ZeroOrderHold  SampleTime=1/10
  Bus Selector : BusSelector  OutputSignals=SL_Slope,SL_Origin
  Bus Selector1 : BusSelector  OutputSignals=Position (inertial)
  Bus Selector3 : BusSelector  OutputSignals=Course
  Chi_d : Subsystem
  Compute crosstrack error : Subsystem
  Constant1 : Constant  Value=Guid.SL.k
  Constant6 : Constant  Value=Guid.SL.chi_inf
  "DerCond " : InportShadow  Port=2
  Goto Tag Visibility : GotoTagVisibility  GotoTag=Vg_prime
  Manual Switch1 : ManualSwitch
  SL.controller : Subsystem
  Selector2 : Selector  InputPortWidth=3  IndexOptions=Index vector (dialog)  Indices=[1 2]  OutputSizes=1
  "Vg " : InportShadow  Port=4
  Vg Estimator : Subsystem
  e_y : Outport
  Vg_hat_SL : Outport  Port=2
  chi_d_SL : Outport  Port=3
  chi_c_SL : Outport  Port=4
  tag scope: Vg_prime=scoped
  wires:
  Compute crosstrack error/2(e_y) -> [e_y]
  Compute crosstrack error/1(chi_q) -> [chi_q]
  [chi_meas] -> SL.controller/1(chi)
  DerCond/1 -> Bus Selector3/1
  [chi_d] -> Manual Switch1/2
  Bus Selector/2 -> Compute crosstrack error/3(SL.Line_Origin)  "<SL_Origin>"
  [e_y] -> Chi_d/1(ey)
  [chi_q] -> Chi_d/2(chi_q)
  Constant6/1 -> Chi_d/3(chi_inf)
  Constant1/1 -> Chi_d/4(k_line)
  Chi_d/1(chi_d) -> [chi_d]
  [chi_d] -> SL.controller/2(chi_d)
  [e_y] -> SL.controller/3(e)
  [Vg_hat] -> SL.controller/4(Vg_hat)
  [chi_q] -> SL.controller/6(chi_q)
  SL.controller/1(chi_c) -> Manual Switch1/1
  GuidData/1 -> Bus Selector/1
  Bus Selector/1 -> Compute crosstrack error/2(SL.Slope)  "<SL_Slope>"
  Manual Switch1/1 -> [chi_c]  "chi_c"
  [chi_d] -> chi_d_SL/1  "chi_d_SL"
  [Vg_hat] -> Vg_hat_SL/1  "Vg_hat_SL"
  [chi_c] -> chi_c_SL/1  "chi_c_SL"
  Bus Selector3/1 -> "10 Hz "/1  "<Course>"
  PlantData/1 -> Bus Selector1/1
  Bus Selector1/1 -> Selector2/1  "<Position (inertial)>"
  Selector2/1 -> 10 Hz/1
  [xy] -> Compute crosstrack error/1(xy)
  [chi_meas] -> Vg Estimator/1(chi_meas)
  [chi_d] -> Vg Estimator/2(chi_d)
  [chi_q] -> Vg Estimator/3(chi_q)
  [e_y] -> Vg Estimator/4(e)
  Vg Estimator/1(Vg_hat) -> [Vg_hat]
  "Vg "/1 -> SL.controller/5(Vg)
  Vg/1 -> Vg Estimator/5(Vg)
  [e_y] -> e_y/1
  Vg_prime/1 -> [Vg_prime]
  "DerCond "/1 -> Vg Estimator/6(DerCond)
  10 Hz/1 -> [xy]
  "10 Hz "/1 -> [chi_meas]
  [chi_meas] -> Compute crosstrack error/4(chi)

== system UAV_sync_unknown_sim/Node 0/VF Approach/PATH MANAGER/Enabled Subsystem ==
  xy : Inport
  Enable : EnablePort
  Bus Creator2 : BusCreator  Inputs=6
  Constant10 : Constant  Value=Path.waypoints
  Constant2 : Constant  Value=Guid.Loiter.R
  Constant3 : Constant  Value=Guid.Loiter.R
  Demux : Demux  Outputs=2
  Path Manager : MATLAB Function  TreatAsAtomicUnit=on
  Selector2 : Selector  InputPortWidth=3  IndexOptions=Index vector (dialog)  Indices=[1 2]  OutputSizes=1
  Stop Simulation : Stop
  GuidData : Outport
  wires:
  Constant10/1 -> Path Manager/1(w)
  Demux/1 -> Path Manager/2(x)
  Path Manager/6(stop_sim) -> Stop Simulation/1
  Selector2/1 -> Demux/1
  Demux/2 -> Path Manager/3(y)
  Constant2/1 -> Path Manager/4(R)
  Bus Creator2/1 -> GuidData/1
  Path Manager/1(flag) -> Bus Creator2/1  "Path flag"
  Path Manager/2(origin) -> Bus Creator2/2  "SL_Origin"
  Path Manager/3(slope) -> Bus Creator2/3  "SL_Slope"
  Path Manager/4(c) -> Bus Creator2/4  "Orbit_C"
  Constant3/1 -> Bus Creator2/5  "Orbit_R"
  Path Manager/5(lambda) -> Bus Creator2/6  "Orbit_j"
  xy/1 -> Selector2/1

== system UAV_sync_unknown_sim/Node 0/VF Approach/PATH MANAGER/Path Following data ==
  Enable : EnablePort
  Bus Creator1 : BusCreator  Inputs=6
  Constant1 : Constant  Value=Guid.SL.Line_Origin
  Constant4 : Constant  Value=Guid.SL.Line_Slope
  Constant5 : Constant  Value=Guid.Loiter.R
  Constant6 : Constant  Value=Guid.Loiter.C
  Constant7 : Constant  Value=Guid.Loiter.j
  Constant8 : Constant  Value=Guid.Strategy
  GuidData : Outport
  wires:
  Constant1/1 -> Bus Creator1/2  "SL_Origin"
  Constant5/1 -> Bus Creator1/5  "Orbit_R"
  Constant7/1 -> Bus Creator1/6  "Orbit_j"
  Constant6/1 -> Bus Creator1/4  "Orbit_C"
  Bus Creator1/1 -> GuidData/1
  Constant8/1 -> Bus Creator1/1  "Path flag"
  Constant4/1 -> Bus Creator1/3  "SL_Slope"

== system UAV_sync_unknown_sim/Node 0/Node 0/Inverse Dynamics Control/Inverse Dynamic 1/Inner Controller ==
  e_x : Inport
  e_y : Inport  Port=2
  e_z : Inport  Port=3
  e_phi : Inport  Port=4
  e_theta : Inport  Port=5
  e_psi : Inport  Port=6
  e_xdot : Inport  Port=7
  e_zdot : Inport  Port=8
  e_phidot : Inport  Port=9
  e_thetadot : Inport  Port=10
  e_psidot : Inport  Port=11
  e_ydot : Inport  Port=12
  Add{1..6} (6 alike) : Sum
  Constant1 : Constant  Value=Derivative_gain_x
  Constant10 : Constant  Value=Proportional_theta
  Constant11 : Constant  Value=Proportional_psi
  Constant12 : Constant  Value=Derivative_gain_psi
  Constant2 : Constant  Value=Derivative_gain_y
  Constant3 : Constant  Value=Proportional_y
  Constant4 : Constant  Value=Derivative_gain_z
  Constant5 : Constant  Value=Proportional_z
  Constant6 : Constant  Value=Derivative_gain_phi
  Constant7 : Constant  Value=Proportional_phi
  Constant8 : Constant  Value=Derivative_gain_theta
  Constant9 : Constant  Value=Proportional_x
  Product{1..12} (12 alike) : Product
  act1 : Outport
  act2 : Outport  Port=2
  act3 : Outport  Port=3
  act4 : Outport  Port=4
  act5 : Outport  Port=5
  act6 : Outport  Port=6
  wires:
  Add5/1 -> act5/1
  Add6/1 -> act6/1
  Add1/1 -> act1/1
  Add3/1 -> act3/1
  Product7/1 -> Add1/2
  Constant9/1 -> Product7/2
  Product1/1 -> Add1/1
  e_x/1 -> Product7/1
  e_xdot/1 -> Product1/2
  Constant1/1 -> Product1/1
  Product3/1 -> Add3/1
  Product9/1 -> Add3/2
  Constant5/1 -> Product9/2
  Constant4/1 -> Product3/1
  e_z/1 -> Product9/1
  Constant7/1 -> Product10/2
  e_phidot/1 -> Product4/2
  Constant6/1 -> Product4/1
  e_phi/1 -> Product10/1
  Product4/1 -> Add4/1
  Product11/1 -> Add5/1
  Constant10/1 -> Product5/2
  e_thetadot/1 -> Product11/2
  Constant8/1 -> Product11/1
  e_theta/1 -> Product5/1
  Product5/1 -> Add5/2
  Constant11/1 -> Product12/2
  Constant12/1 -> Product6/1
  e_psidot/1 -> Product6/2
  Product12/1 -> Add6/2
  e_psi/1 -> Product12/1
  Product6/1 -> Add6/1
  Product10/1 -> Add4/2
  e_zdot/1 -> Product3/2
  e_y/1 -> Product2/2
  Product2/1 -> Add2/1
  Product8/1 -> Add2/2
  Constant2/1 -> Product2/1
  e_ydot/1 -> Product8/1
  Constant3/1 -> Product8/2
  Add2/1 -> act2/1
  Add4/1 -> act4/1

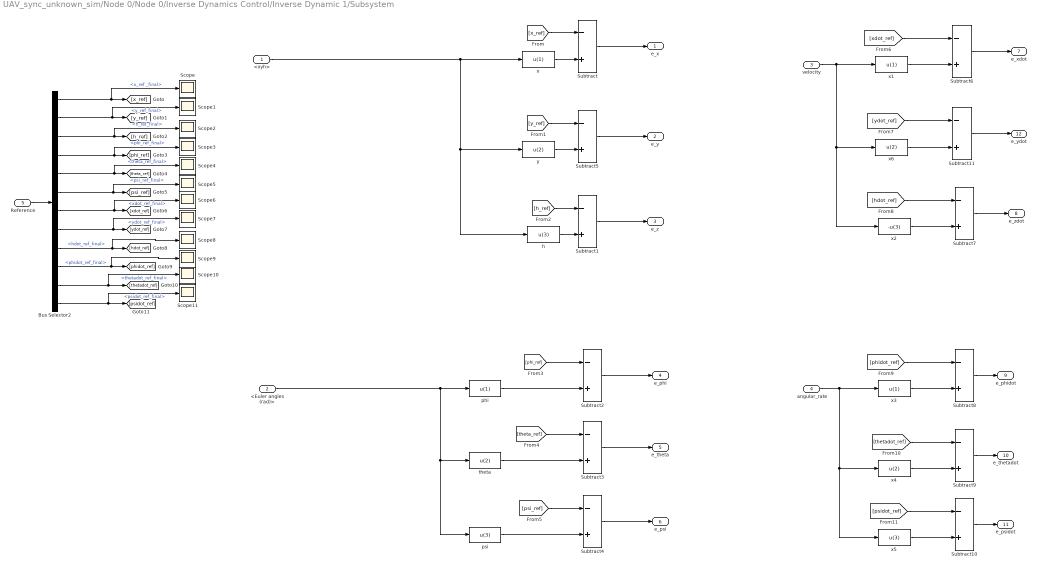
== system UAV_sync_unknown_sim/Node 0/Node 0/Inverse Dynamics Control/Inverse Dynamic 1/Subsystem ==
  <xyh> : Inport
  <Euler angles (rad)> : Inport  Port=2
  velocity : Inport  Port=3
  angular_rate : Inport  Port=4
  Reference : Inport  Port=5
  Bus Selector2 : BusSelector  OutputSignals=x_ref _final,y_ref_final,h_ref_final,phi_ref_final,theta_ref_final,psi_ref_final,xdot_ref_final,ydot_ref_final,hdot_ref_final,phidot_ref_final,thetadot_ref_final,psidot_ref_final
  Scope{,1..11} (12 alike) : Scope
  Subtract{,1..11} (12 alike) : Sum  Inputs=-+
  h : Fcn  Expr=u(3)
  phi : Fcn  Expr=u(1)
  psi : Fcn  Expr=u(3)
  theta : Fcn  Expr=u(2)
  x : Fcn  Expr=u(1)
  x1 : Fcn  Expr=u(1)
  x2 : Fcn  Expr=-u(3)
  x3 : Fcn  Expr=u(1)
  x4 : Fcn  Expr=u(2)
  x5 : Fcn  Expr=u(3)
  x6 : Fcn  Expr=u(2)
  y : Fcn  Expr=u(2)
  e_x : Outport
  e_y : Outport  Port=2
  e_z : Outport  Port=3
  e_phi : Outport  Port=4
  e_theta : Outport  Port=5
  e_psi : Outport  Port=6
  e_xdot : Outport  Port=7
  e_zdot : Outport  Port=8
  e_phidot : Outport  Port=9
  e_thetadot : Outport  Port=10
  e_psidot : Outport  Port=11
  e_ydot : Outport  Port=12
  wires:
  [h_ref] -> Subtract1/1
  h/1 -> Subtract1/2
  <Euler angles (rad)>/1 -> psi/1, theta/1, phi/1
  <xyh>/1 -> h/1, y/1, x/1
  [x_ref] -> Subtract/1
  x/1 -> Subtract/2
  Subtract10/1 -> e_psidot/1
  Subtract9/1 -> e_thetadot/1
  Subtract6/1 -> e_xdot/1
  Subtract5/1 -> e_y/1
  y/1 -> Subtract5/2
  x2/1 -> Subtract7/2
  x1/1 -> Subtract6/2
  velocity/1 -> x6/1, x2/1, x1/1
  Subtract/1 -> e_x/1
  Subtract2/1 -> e_phi/1
  angular_rate/1 -> x3/1, x4/1, x5/1
  x4/1 -> Subtract9/2
  Subtract3/1 -> e_theta/1
  x5/1 -> Subtract10/2
  Subtract4/1 -> e_psi/1
  [xdot_ref] -> Subtract6/1
  [hdot_ref] -> Subtract7/1
  Subtract7/1 -> e_zdot/1
  Subtract8/1 -> e_phidot/1
  Subtract11/1 -> e_ydot/1
  [y_ref] -> Subtract5/1
  Subtract1/1 -> e_z/1
  [ydot_ref] -> Subtract11/1
  x6/1 -> Subtract11/2
  [phidot_ref] -> Subtract8/1
  [thetadot_ref] -> Subtract9/1
  [psidot_ref] -> Subtract10/1
  phi/1 -> Subtract2/2
  x3/1 -> Subtract8/2
  Reference/1 -> Bus Selector2/1
  Bus Selector2/1 -> Scope/1, [x_ref]  "<x_ref _final>"
  Bus Selector2/2 -> Scope1/1, [y_ref]  "<y_ref_final>"
  Bus Selector2/3 -> Scope2/1, [h_ref]  "<h_ref_final>"
  Bus Selector2/4 -> Scope3/1, [phi_ref]  "<phi_ref_final>"
  Bus Selector2/5 -> Scope4/1, [theta_ref]  "<theta_ref_final>"
  Bus Selector2/6 -> Scope5/1, [psi_ref]  "<psi_ref_final>"
  Bus Selector2/7 -> Scope6/1, [xdot_ref]  "<xdot_ref_final>"
  Bus Selector2/8 -> Scope7/1, [ydot_ref]  "<ydot_ref_final>"
  Bus Selector2/9 -> Scope8/1, [hdot_ref]  "<hdot_ref_final>"
  Bus Selector2/12 -> Scope11/1, [psidot_ref]  "<psidot_ref_final>"
  Bus Selector2/10 -> Scope9/1, [phidot_ref]  "<phidot_ref_final>"
  Bus Selector2/11 -> Scope10/1, [thetadot_ref]  "<thetadot_ref_final>"
  theta/1 -> Subtract3/2
  psi/1 -> Subtract4/2
  [phi_ref] -> Subtract2/1
  [theta_ref] -> Subtract3/1
  [psi_ref] -> Subtract4/1

== system UAV_sync_unknown_sim/Node 0/Node 0/Inverse Dynamics Control/Inverse Dynamic 2/Rot_Matrix [3x3] ==
  p : Inport
  q : Inport  Port=2
  r : Inport  Port=3
  Zero : Inport  Port=4
  I1 : Inport  Port=5
  I5 : Inport  Port=6
  I9 : Inport  Port=7
  I3_I7 : Inport  Port=8
  Add : Sum  Inputs=+-
  Add1 : Sum  Inputs=+-
  Gain1 : Gain  Gain=-1
  Gain2 : Gain  Gain=-1
  Gain3 : Gain  Gain=-1
  Product{1..5} (5 alike) : Product
  Reshape : Reshape  OutputDimensionality=Customize  OutputDimensions=[3,3]
  Vector Concatenate : Concatenate  NumInputs=9
  Out1 : Outport
  wires:
  Add/1 -> Gain1/1, Vector Concatenate/2
  Vector Concatenate/1 -> Reshape/1
  Gain3/1 -> Vector Concatenate/3
  Gain2/1 -> Vector Concatenate/8
  I1/1 -> Product3/2
  I9/1 -> Product4/2
  Product2/1 -> Gain3/1, Vector Concatenate/7
  I5/1 -> Product2/2
  Gain1/1 -> Vector Concatenate/4
  Add1/1 -> Vector Concatenate/6, Gain2/1
  r/1 -> Product5/1, Product4/1
  q/1 -> Product2/1
  Zero/1 -> Vector Concatenate/9, Vector Concatenate/5, Vector Concatenate/1
  Reshape/1 -> Out1/1
  p/1 -> Product1/1, Product3/1
  I3_I7/1 -> Product5/2, Product1/2
  Product4/1 -> Add/1
  Product1/1 -> Add/2
  Product5/1 -> Add1/2
  Product3/1 -> Add1/1

== system UAV_sync_unknown_sim/Node 0/Node 0/Inverse Dynamics Control/Inverse Dynamic 2/Trans_Matrix [3x3] ==
  p : Inport
  q : Inport  Port=2
  r : Inport  Port=3
  zero : Inport  Port=4
  M : Inport  Port=5
  Gain2 : Gain  Gain=-1
  Gain3 : Gain  Gain=-1
  Gain4 : Gain  Gain=-1
  Product2 : Product
  Product3 : Product
  Product4 : Product
  Reshape : Reshape  OutputDimensionality=Customize  OutputDimensions=[3,3]
  Vector Concatenate : Concatenate  NumInputs=9
  Out1 : Outport
  wires:
  r/1 -> Product2/1
  q/1 -> Product3/1
  Reshape/1 -> Out1/1
  Product2/1 -> Vector Concatenate/4, Gain4/1
  Vector Concatenate/1 -> Reshape/1
  Product4/1 -> Vector Concatenate/8, Gain2/1
  Gain2/1 -> Vector Concatenate/6
  p/1 -> Product4/1
  M/1 -> Product4/2, Product3/2, Product2/2
  Product3/1 -> Gain3/1, Vector Concatenate/3
  Gain3/1 -> Vector Concatenate/7
  zero/1 -> Vector Concatenate/5, Vector Concatenate/1, Vector Concatenate/9
  Gain4/1 -> Vector Concatenate/2

== system UAV_sync_unknown_sim/Node 0/VF Approach/AUTOPILOT/Low-level Controllers/Get scaling factor ==
  APlane.scaling_speed : Constant  Value=APlane.scaling_speed
  Divide : Product  Inputs=*/
  Saturation : Saturate  UpperLimit=1.67  LowerLimit=0.6
  Scaler : Outport
  wires:
  [Va] -> Divide/2
  Divide/1 -> Saturation/1
  APlane.scaling_speed/1 -> Divide/1
  Saturation/1 -> Scaler/1

== system UAV_sync_unknown_sim/Node 0/VF Approach/AUTOPILOT/Low-level Controllers/Pitch controller ==
  PitchReference : Inport  Unit=deg
  EulerAngles : Inport  Port=2  Unit=deg
  AngularRates : Inport  Port=3  Unit=deg/s
  Scaler : Inport  Port=4
  1/Ctr.Roll.RLL2SRV_TCONST : Gain  Gain=1/Ctr.Roll.RLL2SRV_TCONST
  Angle Conversion1 : aerolibconvert2/Angle Conversion  IU=deg  OU=rad
  Angle Conversion5 : aerolibconvert2/Angle Conversion  IU=deg  OU=rad
  Coordination offset : Subsystem
  Pitch PID : Subsystem
  Rate limiter : Saturate  UpperLimit=Ctr.Pitch.PTCH2SRV_RMAX_UP  LowerLimit=-Ctr.Pitch.PTCH2SRV_RMAX_DN  LinearizeAsGain=off
  Saturation1 : Saturate  UpperLimit=80  LowerLimit=-80
  Selector1 : Selector  InputPortWidth=3  IndexOptions=Index vector (dialog)  Indices=2  OutputSizes=1
  Selector2 : Selector  InputPortWidth=3  IndexOptions=Index vector (dialog)  Indices=1  OutputSizes=1
  Selector3 : Selector  InputPortWidth=3  IndexOptions=Index vector (dialog)  Indices=1  OutputSizes=1
  Selector4 : Selector  InputPortWidth=3  IndexOptions=Index vector (dialog)  Indices=2  OutputSizes=1
  Sum : Sum  Inputs=++|
  Sum1 : Sum  Inputs=|+-
  TRASH : Subsystem  Commented=on
  ElevDemand : Outport
  wires:
  AngularRates/1 -> Selector1/1
  Selector2/1 -> Angle Conversion1/1  "roll_angle"
  EulerAngles/1 -> Selector3/1, Selector2/1, Selector4/1
  Selector1/1 -> Pitch PID/3(Meas_pitch_rate)  "pitch_rate"
  Selector4/1 -> Sum1/2, [pitch_ang]
  PitchReference/1 -> Sum1/1
  Sum/1 -> Pitch PID/1(DesRate)
  Selector3/1 -> Pitch PID/4(Meas_roll_angle)
  Scaler/1 -> Pitch PID/2(Scaler)
  Coordination offset/1(Pitch_rate_correction) -> Sum/1
  Sum1/1 -> 1/Ctr.Roll.RLL2SRV_TCONST/1
  1/Ctr.Roll.RLL2SRV_TCONST/1 -> Rate limiter/1
  Rate limiter/1 -> Sum/2
  [pitch_ang] -> Angle Conversion5/1
  Saturation1/1 -> Coordination offset/2(bank)
  [Va] -> Coordination offset/3(Va)
  Angle Conversion5/1 -> Coordination offset/1(pitch)
  Angle Conversion1/1 -> Saturation1/1
  Pitch PID/1(ElevDemand) -> ElevDemand/1

== system UAV_sync_unknown_sim/Node 0/VF Approach/AUTOPILOT/Low-level Controllers/Roll controller ==
  RollReference : Inport  Unit=deg
  Euler angles : Inport  Port=2  Unit=deg
  AngularRates : Inport  Port=3  Unit=deg/s
  Scaler : Inport  Port=4
  Discrete PID Controller : simulink/Continuous/PID Controller  Controller=PI  Form=Parallel  TimeDomain=Discrete-time  SampleTime=Ctr.TS  IntegratorMethod=Forward Euler  FilterMethod=Forward Euler  ControllerParametersSource=internal  P=1.28067056525733  I=0.869761866515897  D=0  UseFilter=on  N=100  TunerSelectOption=Transfer Function Based (PID Tuner App)  InitialConditionSource=internal  InitialConditionForIntegrator=0  InitialConditionForFilter=0  DifferentiatorICPrevScaledInput=0  ExternalReset=none  TrackingMode=off  Kt=1  LimitOutput=on  UpperSaturationLimit=Ctr.Roll.RLL2SRV_RMAX  LowerSaturationLimit=-Ctr.Roll.RLL2SRV_RMAX  LinearizeAsGain=off  AntiWindupMode=clamping  Kb=1  POutMin=[]  POutMax=[]  IOutMin=[]  IOutMax=[]  DOutMin=[]  DOutMax=[]  NOutMin=[]  NOutMax=[]  SumOutMin=[]  SumOutMax=[]  SaturationOutMin=[]  SaturationOutMax=[]  PParamMin=[]  PParamMax=[]  IParamMin=[]  IParamMax=[]  DParamMin=[]  DParamMax=[]  NParamMin=[]  NParamMax=[]  KbParamMin=[]  KbParamMax=[]  KtParamMin=[]  KtParamMax=[]  KbOutMin=[]  KbOutMax=[]  KtOutMin=[]  KtOutMax=[]  IntegratorOutMin=[]  IntegratorOutMax=[]  FilterOutMin=[]  FilterOutMax=[]  SumI1OutMin=[]  SumI1OutMax=[]  SumI2OutMin=[]  SumI2OutMax=[]  SumI3OutMin=[]  SumI3OutMax=[]  SumI4OutMin=[]  SumI4OutMax=[]  SumDOutMin=[]  SumDOutMax=[]  DifferentiatorOutMin=[]  DifferentiatorOutMax=[]  FilterDiffOutCoefMin=[]  FilterDiffOutCoefMax=[]  ReciprocalOutMin=[]  ReciprocalOutMax=[]  SumDenOutMin=[]  SumDenOutMax=[]  SumNumOutMin=[]  SumNumOutMax=[]  DivideOutMin=[]  DivideOutMax=[]  IntegratorContinuousStateAttributes=''  IntegratorStateMustResolveToSignalObject=off  IntegratorRTWStateStorageClass=Auto  FilterContinuousStateAttributes=''  FilterStateMustResolveToSignalObject=off  FilterRTWStateStorageClass=Auto  ParallelPVariant=InternalParameters  IdealPVariant=Disabled  IVariant=InternalParameters  DVariant=Disabled  IntegratorVariant=Discrete  SatVariant=Enabled  AWVariant=DiscClampingParallel  PCopyVariant=Disabled  TRVariant=Disabled  FdbkBlocksVariant=Forward  IdealPFdbkVariant=Disabled  SatFdbkVariant=Disabled  DerivativeFilterVariant=Disabled  NVariant=Disabled  NCopyVariant=Disabled_SignalSpec  FilterICVariant=Disabled  IntegratorICVariant=InternalICs  ExternalResetVariant=Disabled  TRSumVariant=Passthrough  SumFdbkVariant=Disabled  SumVariant=Sum_PI
  Manual Switch : ManualSwitch  CurrentSetting=0
  Manual Switch1 : ManualSwitch
  OMEGA : Gain  Gain=Ctr.Roll.OMEGA
  Roll Rate Controller : Subsystem
  Roll Rate Controller (simpl. continuous) : Subsystem  Commented=on
  "Scaler " : InportShadow  Port=4
  Scope : Scope  NumInputPorts=2
  Scope1 : Scope
  Selector : Selector  InputPortWidth=3  IndexOptions=Index vector (dialog)  Indices=1  OutputSizes=1
  Selector1 : Selector  InputPortWidth=3  IndexOptions=Index vector (dialog)  Indices=1  OutputSizes=1
  Sum : Sum  Inputs=|+-
  gainsrmax(deg/s) : Saturate  UpperLimit=Ctr.Roll.RLL2SRV_RMAX  LowerLimit=-Ctr.Roll.RLL2SRV_RMAX
  AilDemand : Outport  Unit=deg
  wires:
  RollReference/1 -> Scope/1, Sum/1
  Scaler/1 -> Roll Rate Controller/3(Scaler)  "m/s"
  AngularRates/1 -> Selector1/1
  Euler angles/1 -> Selector/1
  Sum/1 -> OMEGA/1, Discrete PID Controller/1, Scope1/1
  Selector1/1 -> Roll Rate Controller (simpl. continuous)/2(Roll rate), Roll Rate Controller/2(Roll Rate)  "roll_rate"
  Selector/1 -> Scope/2, Sum/2
  Manual Switch/1 -> Roll Rate Controller (simpl. continuous)/1(Roll Rate Error), Roll Rate Controller/1(Desidered rate)  "roll_rate_erorr [deg/s]"
  Manual Switch1/1 -> AilDemand/1
  Roll Rate Controller/1(Ail_dem) -> Manual Switch1/1
  "Scaler "/1 -> Roll Rate Controller (simpl. continuous)/3(Scaler)  "m/s"
  Roll Rate Controller (simpl. continuous)/1(AilDemand) -> Manual Switch1/2
  OMEGA/1 -> gainsrmax(deg/s)/1
  gainsrmax(deg/s)/1 -> Manual Switch/2  "roll_rate_erorr [deg/s]"
  Discrete PID Controller/1 -> Manual Switch/1

== system UAV_sync_unknown_sim/Node 0/VF Approach/AUTOPILOT/Low-level Controllers/Side-slip angle controller ==
  note: - Ctr.Yaw.YAW2SRV_SLIP enables side-slip angle control (disabled)
      | - Ctr.Yaw.YAW2SRV_DAMP enables the yaw angle damping (enabled)
  note: Roll Mixer = Aileron Rudder Interconnect (ARI). Disabled cause it creates an additional roll-yaw cross-coupling.
  note: Roll mixer
  Yaw_rate : Inport
  "Euler angles " : Inport  Port=2
  accel_y : Inport  Port=3
  Scaler : Inport  Port=4
  AilDemand : Inport  Port=5
  Angle Conversion : aerolibconvert2/Angle Conversion  IU=rad  OU=deg
  Coordination offset : Subsystem
  "Ctr.Yaw.KFF_RDDRMIX " : Gain  Gain=-1*Ctr.Yaw.KFF_RDDRMIX
  Ctr.Yaw.YAW2SRV_DAMP : Gain  Gain=Ctr.Yaw.YAW2SRV_DAMP
  Ctr.Yaw.YAW2SRV_INT : Gain  Gain=Ctr.Yaw.YAW2SRV_INT
  Ctr.Yaw.YAW2SRV_SLIP : Gain  Gain=Ctr.Yaw.YAW2SRV_SLIP+0.25
  Discrete-Time Integrator : DiscreteIntegrator  SampleTime=Ctr.TS  UpperSaturationLimit=deg2rad(15)  LowerSaturationLimit=deg2rad(-15)  ICPrevOutput=DiscIntNeverNeededParam  ICPrevScaledInput=DiscIntNeverNeededParam
  Gain4 : Gain  Gain=-1
  High-Pass Filter : Subsystem
  Math Function : Math  Operator=square  SaturateOnIntegerOverflow=on
  Product : Product
  Saturation : Saturate  UpperLimit=45  LowerLimit=-45
  Scope : Scope
  Scope1 : Scope
  Scope2 : Scope
  Selector1 : Selector  InputPortWidth=3  IndexOptions=Index vector (dialog)  Indices=1  OutputSizes=1
  Selector4 : Selector  InputPortWidth=3  IndexOptions=Index vector (dialog)  Indices=2  OutputSizes=1
  Selector5 : Selector  InputPortWidth=3  IndexOptions=Index vector (dialog)  Indices=3  OutputSizes=1
  Sum : Sum  Inputs=|+-
  Sum1 : Sum  Inputs=|+-
  Sum2 : Sum  Inputs=|+-
  Sum3 : Sum  Inputs=|++
  on/off : Gain
  RudderDemand : Outport
  wires:
  Ctr.Yaw.YAW2SRV_SLIP/1 -> Sum/1
  Yaw_rate/1 -> Selector5/1
  Sum1/1 -> High-Pass Filter/1(In)  "r_err"
  High-Pass Filter/1(Out) -> Scope2/1, Sum2/2, Sum/2
  Sum/1 -> Ctr.Yaw.YAW2SRV_INT/1
  Ctr.Yaw.YAW2SRV_INT/1 -> Discrete-Time Integrator/1
  Discrete-Time Integrator/1 -> Sum2/1
  Sum2/1 -> Ctr.Yaw.YAW2SRV_DAMP/1
  Ctr.Yaw.YAW2SRV_DAMP/1 -> Product/1
  Scaler/1 -> Math Function/1
  Math Function/1 -> Product/2
  Product/1 -> Gain4/1
  Selector5/1 -> Sum1/1
  Angle Conversion/1 -> Sum3/1
  Gain4/1 -> Angle Conversion/1
  Sum3/1 -> Saturation/1
  "Ctr.Yaw.KFF_RDDRMIX "/1 -> Sum3/2
  Saturation/1 -> on/off/1
  AilDemand/1 -> "Ctr.Yaw.KFF_RDDRMIX "/1
  "Euler angles "/1 -> Selector1/1
  Coordination offset/1(yaw_rate_correction) -> Sum1/2
  Selector1/1 -> Coordination offset/1(Bank)
  accel_y/1 -> Selector4/1
  Selector4/1 -> Ctr.Yaw.YAW2SRV_SLIP/1, Scope/1
  on/off/1 -> RudderDemand/1, Scope1/1
